simulink model "PV_MPPT_C2000_Host"  (R2018b)
settings: Solver=VariableStepAuto  StartTime=0.0  StopTime=inf  RelTol=1e-3
PreLoadFcn:
  | load('EmulatedPV_LowPowerData.mat');
  | 
  | numIrr = 6;
  | ArrayPower = ArrayCurrent.*ArrayVoltage;
InitFcn:
  | IQ8 = 256;
  | IQ13 = 8192;
  | IQ15 = 32768;
  | IQ24 = 16777216;
  | 
  | InvFreq = 50;
  | 
  | Tdata = 0.05;
  | Tcontrol = 1e-4;
undefined symbols (not defined in the file): ArrayVoltage, DiscIntNeverNeededParam, serial
libraries: instrumentlib x3
settings Model: Creator=jlesage  LastModifiedBy=jlesage
settings DebuggingCC: LibraryContextMissingDiagnostic=none
settings SFSimCC: SimUseLocalCustomCode=off
settings RTWCC: RTWUseLocalCustomCode=off

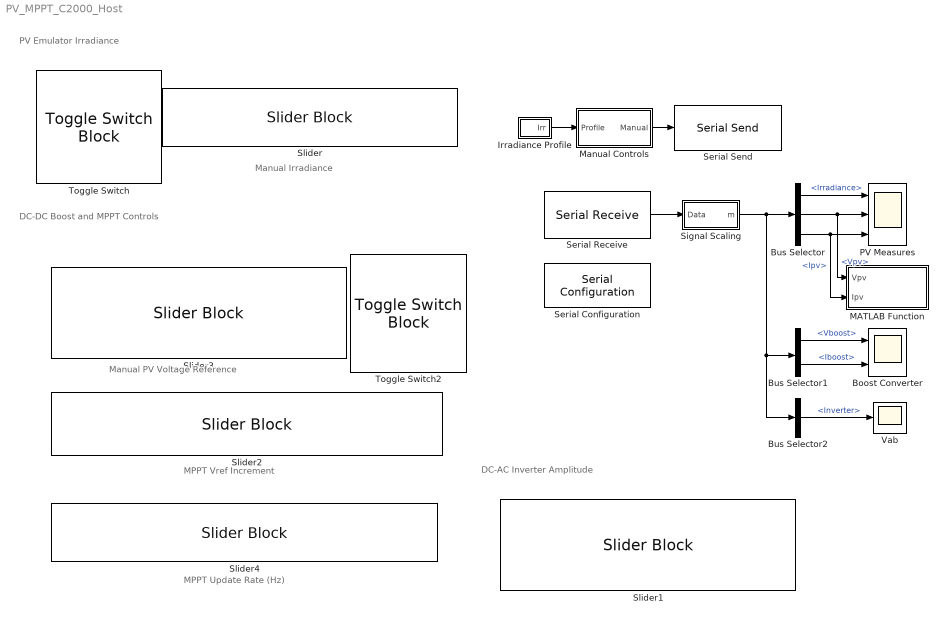
== system PV_MPPT_C2000_Host ==
  note: DC-AC Inverter Amplitude
  note: MPPT Vref Increment
  note: DC-DC Boost and MPPT Controls
  note: Manual Irradiance
  note: PV Emulator Irradiance
  note: Manual PV Voltage Reference
  note: MPPT Update Rate (Hz)
  Boost Converter : Scope  NumInputPorts=2
  Bus Selector : BusSelector  OutputSignals=PV.Irradiance,PV.Vpv,PV.Ipv
  Bus Selector1 : BusSelector  OutputSignals=Boost.Vboost,Boost.Iboost
  Bus Selector2 : BusSelector  OutputSignals=Inverter
  Irradiance Profile : Subsystem
  MATLAB Function : MATLAB Function  TreatAsAtomicUnit=on  SystemSampleTime=0.05
  Manual Controls : Subsystem
  PV Measures : Scope  NumInputPorts=3
  Serial Configuration : instrumentlib/Serial Configuration  Priority=-200000  ComPortMenu=<Please select a port...>  ComPort=COM6  ObjConstructor=serial('COM6');  BaudRate=9600  DataBits=8  Parity=none  StopBits=1  FlowControl=none  Timeout=10  ByteOrder=LittleEndian
  Serial Receive : instrumentlib/Serial Receive  ComPortMenu=<Please select a port...>  ComPort=COM6  ObjConstructor=serial('COM6');  Header=S  Terminator=E  DataSize="[7  1]"  DataType=uint16  EnableBlockingMode=on  ActionDataUnavailable=Output last received value  CustomValue=0  SampleTime=0.05
  Serial Send : instrumentlib/Serial Send  ComPortMenu=<Please select a port...>  ComPort=COM6  ObjConstructor=serial('COM6');  Header=B  Terminator=T  EnableBlockingMode=off
  Signal Scaling : Subsystem
  Slider : SliderBlock  WebBlockId=167  ScaleMax=0.5  TickInterval=0.10000000000000001
  Slider1 : SliderBlock  WebBlockId=168  ScaleMax=1  TickInterval=0.10000000000000001
  Slider2 : SliderBlock  WebBlockId=169  ScaleMax=0.5  TickInterval=0.10000000000000001
  Slider3 : SliderBlock  WebBlockId=170  ScaleMin=1  ScaleMax=10  TickInterval=1
  Slider4 : SliderBlock  WebBlockId=166  ScaleMin=25  ScaleMax=250  TickInterval=25
  Toggle Switch : ToggleSwitchBlock  WebBlockId=164  LabelPosition=Hide
      settings: Values={{'Use Profile', 'Set Irradiance'}, [0 1]}
  Toggle Switch2 : ToggleSwitchBlock  WebBlockId=165  LabelPosition=Hide
      settings: Values={{'Manual Vref', 'Enable MPPT'}, [0 1]}
  Vab : Scope
  wires:
  Bus Selector/1 -> PV Measures/1  "<Irradiance>"
  Bus Selector/2 -> MATLAB Function/1(Vpv), PV Measures/2  "<Vpv>"
  Bus Selector/3 -> MATLAB Function/2(Ipv), PV Measures/3  "<Ipv>"
  Bus Selector1/1 -> Boost Converter/1  "<Vboost>"
  Bus Selector1/2 -> Boost Converter/2  "<Iboost>"
  Serial Receive/1 -> Signal Scaling/1(Data)
  Signal Scaling/1(m) -> Bus Selector2/1, Bus Selector1/1, Bus Selector/1
  Manual Controls/1(Manual) -> Serial Send/1
  Bus Selector2/1 -> Vab/1  "<Inverter>"
  Irradiance Profile/1(Irr) -> Manual Controls/1(Profile)

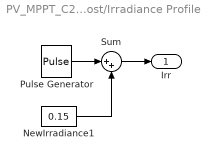
== system PV_MPPT_C2000_Host/Irradiance Profile ==
  NewIrradiance1 : Constant  Value=0.15  OutDataTypeStr=single
  Pulse Generator : DiscretePulseGenerator  PulseType=Time based  Amplitude=0.1  Period=10  PulseWidth=50
  Sum : Sum  Inputs=|++
  Irr : Outport
  wires:
  NewIrradiance1/1 -> Sum/2
  Sum/1 -> Irr/1
  Pulse Generator/1 -> Sum/1

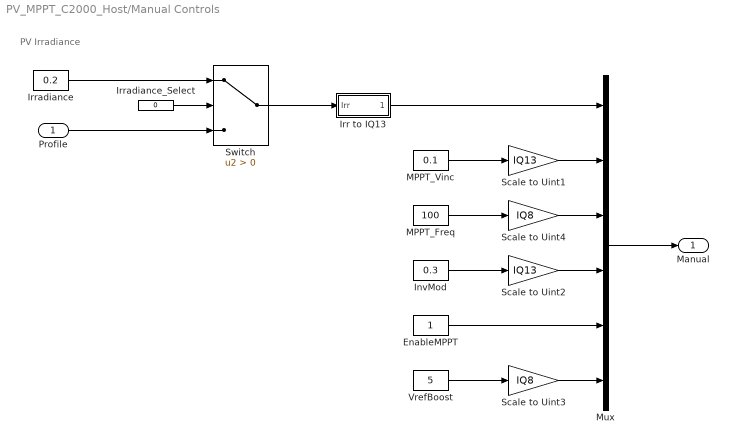
== system PV_MPPT_C2000_Host/Manual Controls ==
  note: PV Irradiance
  Profile : Inport
  EnableMPPT : Constant  OutDataTypeStr=uint16
  InvMod : Constant  Value=0.3  OutDataTypeStr=single
  Irr to IQ13 : Subsystem
  Irradiance : Constant  Value=0.2  OutDataTypeStr=single
  Irradiance_Select : Constant  Value=0  OutDataTypeStr=single
  MPPT_Freq : Constant  Value=100  OutDataTypeStr=single
  MPPT_Vinc : Constant  Value=0.1  OutDataTypeStr=single
  Mux : Mux  Inputs=6
  Scale to Uint1 : Gain  Gain=IQ13  OutDataTypeStr=uint16
  Scale to Uint2 : Gain  Gain=IQ13  OutDataTypeStr=uint16
  Scale to Uint3 : Gain  Gain=IQ8  OutDataTypeStr=uint16
  Scale to Uint4 : Gain  Gain=IQ8  OutDataTypeStr=uint16
  Switch : Switch  Criteria=u2 > Threshold
  VrefBoost : Constant  Value=5  OutDataTypeStr=single
  Manual : Outport
  wires:
  Irradiance/1 -> Switch/1
  Scale to Uint1/1 -> Mux/2
  MPPT_Vinc/1 -> Scale to Uint1/1
  Mux/1 -> Manual/1
  InvMod/1 -> Scale to Uint2/1
  Irradiance_Select/1 -> Switch/2
  Switch/1 -> Irr to IQ13/1(Irr)
  Irr to IQ13/1(Uint16) -> Mux/1
  Profile/1 -> Switch/3
  Scale to Uint2/1 -> Mux/4
  MPPT_Freq/1 -> Scale to Uint4/1
  EnableMPPT/1 -> Mux/5
  VrefBoost/1 -> Scale to Uint3/1
  Scale to Uint3/1 -> Mux/6
  Scale to Uint4/1 -> Mux/3

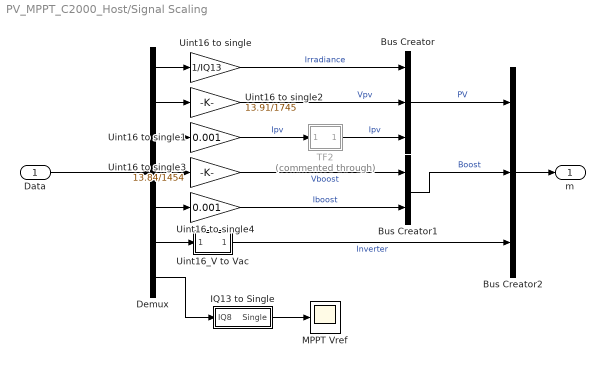
== system PV_MPPT_C2000_Host/Signal Scaling ==
  Data : Inport
  Bus Creator : BusCreator  Inputs=3
  Bus Creator1 : BusCreator  Inputs=2
  Bus Creator2 : BusCreator  Inputs=3
  Demux : Demux  Outputs=7
  IQ13 to Single : Subsystem
  MPPT Vref : Scope
  TF2 : Subsystem  Commented=through  mask{Tf=0.1}
      mask prompts: Tf "Filter Time Constant"
      mask Display: fprintf('1\n------------\n(1 + s Ta3)');
  Uint16 to single : Gain  Gain=1/IQ13  OutDataTypeStr=single
  Uint16 to single1 : Gain  Gain=0.001  OutDataTypeStr=single
  Uint16 to single2 : Gain  Gain=13.91/1745  OutDataTypeStr=single
  Uint16 to single3 : Gain  Gain=13.84/1454  OutDataTypeStr=single
  Uint16 to single4 : Gain  Gain=0.001  OutDataTypeStr=single
  Uint16_V to Vac : Subsystem
  m : Outport
  wires:
  Data/1 -> Demux/1
  Demux/2 -> Uint16 to single2/1
  Demux/1 -> Uint16 to single/1
  Demux/3 -> Uint16 to single1/1
  Demux/5 -> Uint16 to single4/1
  Demux/4 -> Uint16 to single3/1
  Uint16 to single1/1 -> TF2/1(In1)  "Ipv"
  Uint16 to single3/1 -> Bus Creator1/1  "Vboost"
  Uint16_V to Vac/1(Vac) -> Bus Creator2/3  "Inverter"
  Demux/6 -> Uint16_V to Vac/1(A7)
  Demux/7 -> IQ13 to Single/1(IQ8)
  Uint16 to single2/1 -> Bus Creator/2  "Vpv"
  Uint16 to single/1 -> Bus Creator/1  "Irradiance"
  Uint16 to single4/1 -> Bus Creator1/2  "Iboost"
  Bus Creator/1 -> Bus Creator2/1  "PV"
  Bus Creator1/1 -> Bus Creator2/2  "Boost"
  Bus Creator2/1 -> m/1
  IQ13 to Single/1(Single) -> MPPT Vref/1
  TF2/1(Out1) -> Bus Creator/3  "Ipv"

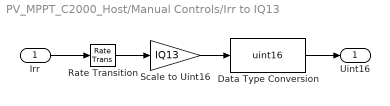
== system PV_MPPT_C2000_Host/Manual Controls/Irr to IQ13 ==
  Irr : Inport
  Data Type Conversion : DataTypeConversion  OutDataTypeStr=uint16
  Rate Transition : RateTransition  InitialCondition=0.3  OutPortSampleTime=Tdata
  Scale to Uint16 : Gain  Gain=IQ13  OutDataTypeStr=single
  Uint16 : Outport
  wires:
  Rate Transition/1 -> Scale to Uint16/1
  Data Type Conversion/1 -> Uint16/1
  Irr/1 -> Rate Transition/1
  Scale to Uint16/1 -> Data Type Conversion/1

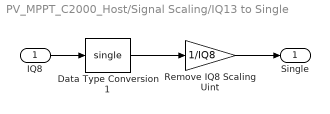
== system PV_MPPT_C2000_Host/Signal Scaling/IQ13 to Single ==
  IQ8 : Inport
  Data Type Conversion1 : DataTypeConversion  OutDataTypeStr=single
  Remove IQ8 Scaling Uint : Gain  Gain=1/IQ8  OutDataTypeStr=single
  Single : Outport
  wires:
  Data Type Conversion1/1 -> Remove IQ8 Scaling Uint/1
  IQ8/1 -> Data Type Conversion1/1
  Remove IQ8 Scaling Uint/1 -> Single/1

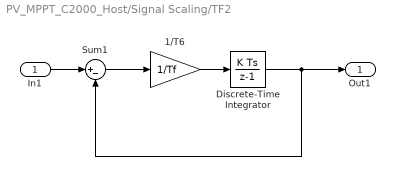
== system PV_MPPT_C2000_Host/Signal Scaling/TF2 ==
  In1 : Inport
  1/T6 : Gain  Gain=1/Tf
  Discrete-Time Integrator : DiscreteIntegrator  SampleTime=-1  ICPrevOutput=DiscIntNeverNeededParam  ICPrevScaledInput=DiscIntNeverNeededParam
  Sum1 : Sum  Inputs=|+-
  Out1 : Outport
  wires:
  Sum1/1 -> 1/T6/1
  Discrete-Time Integrator/1 -> Sum1/2, Out1/1
  In1/1 -> Sum1/1
  1/T6/1 -> Discrete-Time Integrator/1

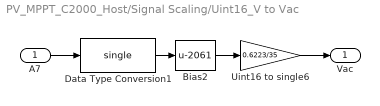
== system PV_MPPT_C2000_Host/Signal Scaling/Uint16_V to Vac ==
  A7 : Inport
  Bias2 : Bias  Bias=-2061
  Data Type Conversion1 : DataTypeConversion  OutDataTypeStr=single
  Uint16 to single6 : Gain  Gain=0.6223/35  OutDataTypeStr=single
  Vac : Outport
  wires:
  Uint16 to single6/1 -> Vac/1
  A7/1 -> Data Type Conversion1/1
  Data Type Conversion1/1 -> Bias2/1
  Bias2/1 -> Uint16 to single6/1

== matlab function PV_MPPT_C2000_Host/MATLAB Function ==
  settings: updateMethod=DISCRETE
  data: Vpv input; Ipv input; ArrayPower parameter; ArrayVoltage parameter; numIrr parameter
function plotPower(Vpv,Ipv, ArrayPower,ArrayVoltage, numIrr)

    persistent irrPlot powerPlot
%     coder.extrinsic('legend');
        
    if isempty(irrPlot)
        
        idx = 1:find(ArrayPower(:,numIrr) > 0,1,'last')+2;
                        
        figure(1);
        irrPlot = plot(ArrayVoltage(idx),ArrayPower(idx,1:numIrr)); hold on;
        grid on;
        
        xlabel('PV Voltage [V]');
        ylabel('PV Power [W]');
        title('PV Power Output');
        
        powerPlot = plot(Vpv,Vpv*Ipv,'ro'); 
%         legend('50 W/m^2','100 W/m^2','150 W/m^2','200 W/m^2',...
%             '250 W/m^2','300 W/m^2','PV Power');
        hold off;
        
    else 
        set(powerPlot,'XData',Vpv,'YData',Vpv*Ipv);
    end
    
end
